simulink model "Homing"  (R2025b)
settings: Solver=FixedStepAuto  StartTime=0.0  StopTime=inf  FixedStep=Ts  RelTol=1e-3
model workspace (MATLAB code in the model file):
  | tgName = 'performance4';
values from neighbouring files (symbols this model uses):
  data = rtRun.export    [postProcess.m]
  Ts = 0.001    [initHoming.m]
undefined symbols (not defined in the file or in its folder): drawWire_m, drawWire_mpers, linearPower_W, netForce_N
libraries: slrealtimeethercatlib x11, slrealtimeloglib x3, simulink x3, eeGeneralControl x3, slrealtimeutilitieslib x2, dspstat3 x2, slrealtimeptplib x1, dspsigops x1
settings Model: Creator=Wave User  LastModifiedBy=bosmab
settings SolverCC: ConcurrentTasks=on  PositivePriorityOrder=on
settings OptimizationCC: BlockReduction=off  OptimizeBlockIOStorage=off
settings DebuggingCC: TasksWithSamePriorityMsg=none
settings HardwareCC: ProdBitPerLong=64.0  ProdLongLongMode=on  ProdHWDeviceType=Intel->x86-64 (Linux 64)
settings RTWCC: SystemTargetFile=speedgoat.tlc  TemplateMakefile=slrealtime_default_tmf  RTWVerbose=off  Toolchain=Simulink Real-Time Toolchain  BuildConfiguration=Faster Runs  CodeExecutionProfiling=on  TargetLang=C++  Description=Speedgoat Real-Time Target Machine
settings SimulinkRealTimeTargetCC: SLRTFileLogMaxRuns=1.0  ExtModeMaxTrigDuration=10.0  ExtModeStaticAllocSize=1000000.0  ExtModeTransport=0.0  MultiwordLength=2048.0  DynamicStringBufferSize=256.0  PreserveMATLABNamespacesInGeneratedCode=on  SubcomponentCodeInterfacePackaging=Reusable function  InstructionSetFMA=off  LogToMDFFile=off

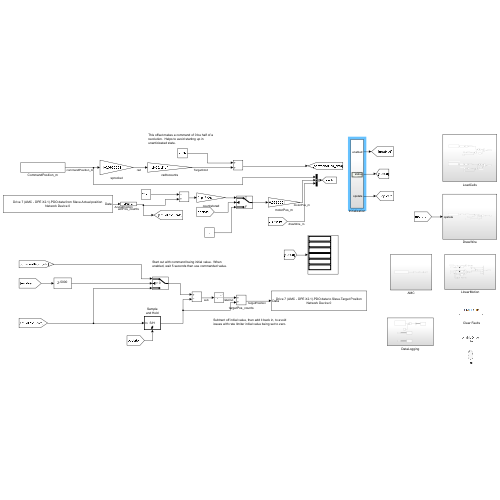
[thumbnail: Simulink's stored preview of the top-level diagram]
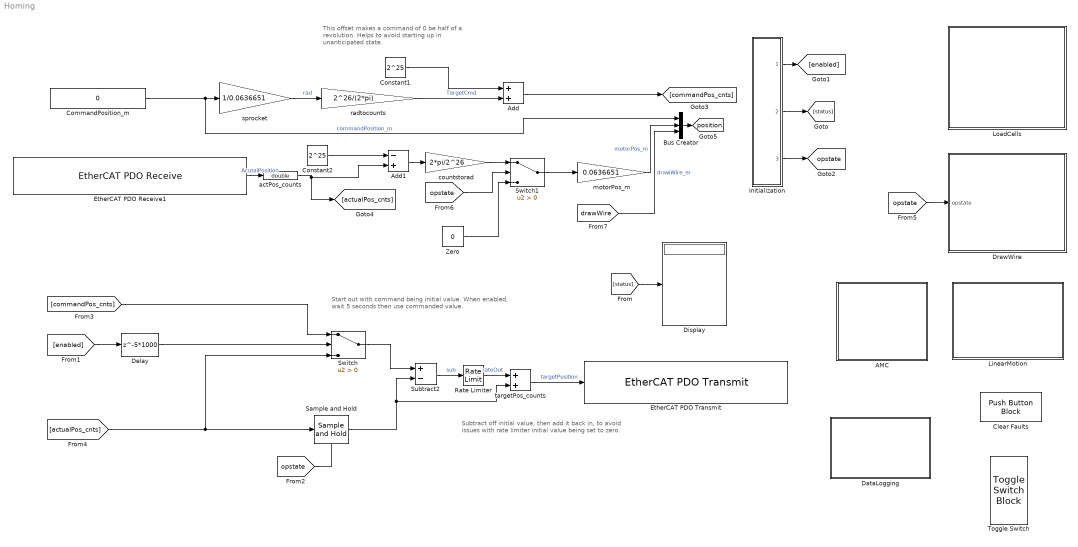
== system Homing ==
  note: Start out with command being initial value. When enabled, wait 5 seconds then use commanded value.
  note: This offset makes a command of 0 be half of a revolution. Helps to avoid starting up in unanticipated state.
  note: Subtract off initial value, then add it back in, to avoid issues with rate limiter initial value being set to zero.
  AMC : Subsystem
  Add : Sum
  Add1 : Sum  Inputs=-+
  Bus Creator : BusCreator  Inputs=3
  Clear Faults : PushButtonBlock  ButtonText=Clear Faults  IconOnColor=[0.0, 0.39215686274509803, 0.0]  IconOffColor=[0.0, 1.0, 0.0]  OffValue=0.000000
  CommandPosition_m : Constant  Value=0  OutDataTypeStr=double
  Constant1 : Constant  Value=2^25  OutDataTypeStr=int32
  Constant2 : Constant  Value=2^25  OutDataTypeStr=double
  DataLogging : Subsystem
  Delay : Delay  DelayLength=5*1000
  Display : Display
  DrawWire : Subsystem
  EtherCAT PDO Receive1 : slrealtimeethercatlib/EtherCAT PDO Receive  Priority=2  sig_name=Drive 7 (AMC - DPE X2.1).PDO data from Slave.Actual position  sig_offset=592  sig_type=int32  type_size=32  sig_dim=1  device_id=0  sample_time=0.001000
  EtherCAT PDO Transmit : slrealtimeethercatlib/EtherCAT PDO Transmit  Priority=3  sig_name=Drive 7 (AMC - DPE X2.1).PDO data to Slave.Target Position  sig_offset=592  sig_type=int32  type_size=32  sig_dim=1  device_id=0  sample_time=0.001000
  Initialization : Subsystem
  LinearMotion : Subsystem
  LoadCells : Subsystem
  Rate Limiter : RateLimiter  RisingSlewLimit=1e6  FallingSlewLimit=-1e6  SampleTimeMode=inherited
  Sample and Hold : dspsigops/Sample and Hold  trig=Rising edge  initCond=0  latchinput=off
  Subtract2 : Sum  Inputs=+-
  Switch : Switch  Criteria=u2 > Threshold  SaturateOnIntegerOverflow=off  InputSameDT=off
  Switch1 : Switch  Criteria=u2 > Threshold  SaturateOnIntegerOverflow=off  InputSameDT=off
  Toggle Switch : ToggleSwitchBlock
  Zero : Constant  Value=0  OutDataTypeStr=Inherit: Inherit via back propagation
  actPos_counts : DataTypeConversion  OutDataTypeStr=double  SaturateOnIntegerOverflow=off  RndMeth=Floor
  countstorad : Gain  Gain=2*pi/2^26  OutDataTypeStr=double
  motorPos_m : Gain  Gain=0.0636651
  radtocounts : Gain  Gain=2^26/(2*pi)  OutDataTypeStr=int32
  sprocket : Gain  Gain=1/0.0636651
  targetPos_counts : Sum  OutDataTypeStr=int32
  tag scope: opstate=global, position=global
  wires:
  Sample and Hold/1 -> Subtract2/2, targetPos_counts/2
  Subtract2/1 -> Rate Limiter/1  "sub"
  Rate Limiter/1 -> targetPos_counts/1  "rateOut"
  targetPos_counts/1 -> EtherCAT PDO Transmit/1  "targetPosition"
  Delay/1 -> Switch/2
  Switch/1 -> Subtract2/1
  [enabled] -> Delay/1
  CommandPosition_m/1 -> Bus Creator/1, sprocket/1  "commandPosition_m"
  sprocket/1 -> radtocounts/1  "rad"
  countstorad/1 -> Switch1/1
  motorPos_m/1 -> Bus Creator/2  "motorPos_m"
  Constant1/1 -> Add/1
  radtocounts/1 -> Add/2  "TargetCmd"
  Add/1 -> [commandPos_cnts]
  EtherCAT PDO Receive1/1 -> actPos_counts/1  "AcutalPosition"
  Constant2/1 -> Add1/1
  Add1/1 -> countstorad/1
  [status] -> Display/1
  Initialization/2(status) -> [status]
  Initialization/1(enabled) -> [enabled]
  Initialization/3(opstate) -> [opstate]
  [opstate] -> Sample and Hold/Trigger
  [commandPos_cnts] -> Switch/1
  [actualPos_cnts] -> Switch/3, Sample and Hold/1
  [opstate] -> DrawWire/1(opstate)
  Zero/1 -> Switch1/3
  [opstate] -> Switch1/2
  Switch1/1 -> motorPos_m/1
  Bus Creator/1 -> [position]
  [drawWire] -> Bus Creator/3  "drawWire_m"
  actPos_counts/1 -> [actualPos_cnts], Add1/2

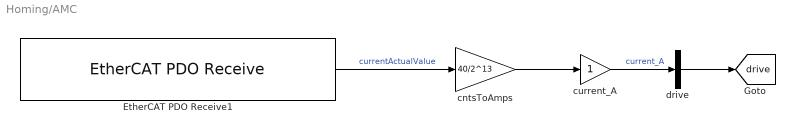
== system Homing/AMC ==
  EtherCAT PDO Receive1 : slrealtimeethercatlib/EtherCAT PDO Receive  Priority=2  sig_name=Drive 7 (AMC - DPE X2.1).PDO data from Slave.Actual Current  sig_offset=656  sig_type=int16  type_size=16  sig_dim=1  device_id=0  sample_time=0.001000
  cntsToAmps : Gain  Gain=40/2^13  OutDataTypeStr=double
  current_A : Gain  OutDataTypeStr=double
  drive : BusCreator  Inputs=1
  tag scope: drive=global
  wires:
  EtherCAT PDO Receive1/1 -> cntsToAmps/1  "currentActualValue"
  drive/1 -> [drive]
  current_A/1 -> drive/1  "current_A"
  cntsToAmps/1 -> current_A/1

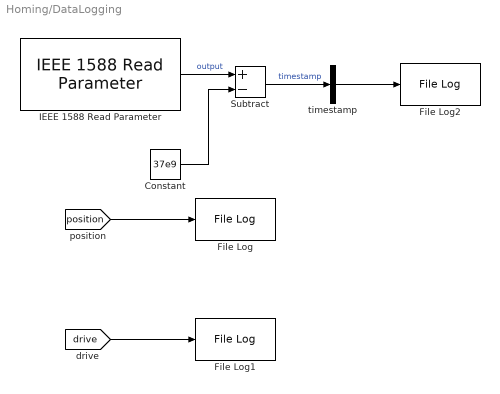
== system Homing/DataLogging ==
  Constant : Constant  Value=37e9  OutDataTypeStr=double
  File Log : slrealtimeloglib/File Log  decimation=1  inputProcessing=Elements as channels (sample based)
  File Log1 : slrealtimeloglib/File Log  decimation=1  inputProcessing=Elements as channels (sample based)
  File Log2 : slrealtimeloglib/File Log  decimation=1  inputProcessing=Elements as channels (sample based)
  IEEE 1588 Read Parameter : slrealtimeptplib/IEEE 1588 Read Parameter  Priority=1  ID=1  param=1. System time (nanosecond)  sample_time=Ts
  Subtract : Sum  Inputs=+-  OutDataTypeStr=double
  timestamp : BusCreator  Inputs=timestamp
  wires:
  [position] -> File Log/1
  [drive] -> File Log1/1
  IEEE 1588 Read Parameter/1 -> Subtract/1  "output"
  Constant/1 -> Subtract/2
  Subtract/1 -> timestamp/1  "timestamp"
  timestamp/1 -> File Log2/1

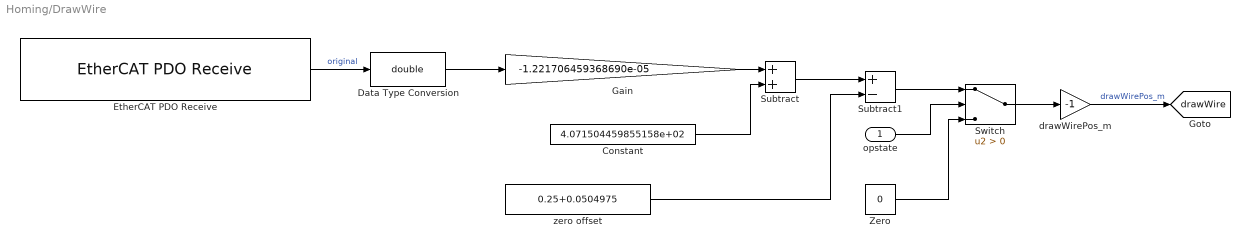
== system Homing/DrawWire ==
  opstate : Inport
  Constant : Constant  Value=4.071504459855158e+02
  Data Type Conversion : DataTypeConversion  OutDataTypeStr=double  SaturateOnIntegerOverflow=off  RndMeth=Floor
  EtherCAT PDO Receive : slrealtimeethercatlib/EtherCAT PDO Receive  Priority=2  sig_name=Term 9 (EL5002).SSI Inputs Channel 1.Counter value  sig_offset=1216  sig_type=uint32  type_size=32  sig_dim=1  device_id=0  sample_time=0.001000
  Gain : Gain  Gain=-1.221706459368690e-05  OutDataTypeStr=double
  Subtract : Sum
  Subtract1 : Sum  Inputs=+-
  Switch : Switch  Criteria=u2 > Threshold  SaturateOnIntegerOverflow=off  InputSameDT=off
  Zero : Constant  Value=0  OutDataTypeStr=Inherit: Inherit via back propagation
  drawWirePos_m : Gain  Gain=-1
  zero offset : Constant  Value=0.25+0.0504975
  tag scope: drawWire=global
  wires:
  Gain/1 -> Subtract/1
  Subtract/1 -> Subtract1/1
  zero offset/1 -> Subtract1/2
  EtherCAT PDO Receive/1 -> Data Type Conversion/1  "original"
  drawWirePos_m/1 -> [drawWire]  "drawWirePos_m"
  Constant/1 -> Subtract/2
  Data Type Conversion/1 -> Gain/1
  Subtract1/1 -> Switch/1
  opstate/1 -> Switch/2
  Switch/1 -> drawWirePos_m/1
  Zero/1 -> Switch/3

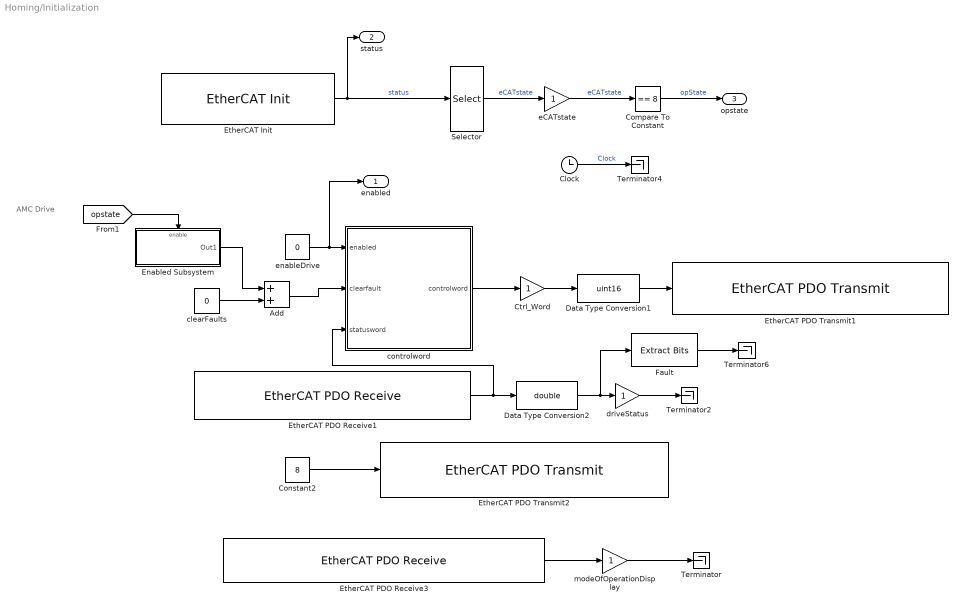
== system Homing/Initialization ==
  note: AMC Drive
  Add : Sum
  Clock : Clock
  Compare To Constant : simulink/Logic and Bit Operations/Compare To Constant  relop===  const=8  OutDataTypeStr=boolean
  Constant2 : Constant  Value=8  OutDataTypeStr=uint16
  Ctrl_Word : Gain
  Data Type Conversion1 : DataTypeConversion  OutDataTypeStr=uint16  SaturateOnIntegerOverflow=off  RndMeth=Floor
  Data Type Conversion2 : DataTypeConversion  OutDataTypeStr=double  SaturateOnIntegerOverflow=off  RndMeth=Floor
  Enabled Subsystem : Subsystem  TreatAsAtomicUnit=on
  EtherCAT Init : slrealtimeethercatlib/EtherCAT Init  Priority=0  config_file=C:\Software\LUPA\Simulink\EtherCAT\LUPAxml.xml  device_id=0  portnum=1  initstate=2  dctuning=0  enaDebug=0  logFile='c:\dbglog.txt'  sample_time=0.001000  DCMode=2
  EtherCAT PDO Receive1 : slrealtimeethercatlib/EtherCAT PDO Receive  Priority=2  sig_name=Drive 7 (AMC - DPE X2.1).PDO data from Slave.Status Word  sig_offset=576  sig_type=uint16  type_size=16  sig_dim=1  device_id=0  sample_time=0.001000
  EtherCAT PDO Receive3 : slrealtimeethercatlib/EtherCAT PDO Receive  Priority=2  sig_name=Drive 7 (AMC - DPE X2.1).PDO data from Slave.Mode Of Operation Display  sig_offset=704  sig_type=uint16  type_size=16  sig_dim=1  device_id=0  sample_time=0.001000
  EtherCAT PDO Transmit1 : slrealtimeethercatlib/EtherCAT PDO Transmit  Priority=3  sig_name=Drive 7 (AMC - DPE X2.1).PDO data to Slave.Control Word  sig_offset=576  sig_type=uint16  type_size=16  sig_dim=1  device_id=0  sample_time=0.001000
  EtherCAT PDO Transmit2 : slrealtimeethercatlib/EtherCAT PDO Transmit  Priority=3  sig_name=Drive 7 (AMC - DPE X2.1).PDO data to Slave.Modes Of Operation  sig_offset=688  sig_type=uint16  type_size=16  sig_dim=1  device_id=0  sample_time=0.001000
  Fault : simulink/Logic and Bit Operations/Extract Bits  bitsToExtract=Range of bits  numBits=8  bitIdxRange=[3]  outScalingMode=Preserve fixed-point scaling
  Selector : Selector  InputPortWidth=6  IndexOptions=Index vector (dialog)  Indices=2  OutputSizes=1
  Terminator{,2,4,6} (4 alike) : Terminator
  clearFaults : Constant  Value=0
  controlword : MATLAB Function  TreatAsAtomicUnit=on
  driveStatus : Gain
  eCATstate : Gain  OutDataTypeStr=double
  enableDrive : Constant  Value=0
  modeOfOperationDisplay : Gain  OutDataTypeStr=double
  enabled : Outport
  status : Outport  Port=2
  opstate : Outport  Port=3
  wires:
  Ctrl_Word/1 -> Data Type Conversion1/1
  enableDrive/1 -> enabled/1, controlword/1(enabled)
  Constant2/1 -> EtherCAT PDO Transmit2/1
  controlword/1(controlword) -> Ctrl_Word/1
  Data Type Conversion2/1 -> Fault/1, driveStatus/1
  EtherCAT PDO Receive1/1 -> Data Type Conversion2/1, controlword/3(statusword)
  Data Type Conversion1/1 -> EtherCAT PDO Transmit1/1
  clearFaults/1 -> Add/2
  driveStatus/1 -> Terminator2/1
  Fault/1 -> Terminator6/1
  Clock/1 -> Terminator4/1  "Clock"
  EtherCAT Init/1 -> status/1, Selector/1  "status"
  eCATstate/1 -> Compare To Constant/1  "eCATstate"
  Selector/1 -> eCATstate/1  "eCATstate"
  Compare To Constant/1 -> opstate/1  "opState"
  EtherCAT PDO Receive3/1 -> modeOfOperationDisplay/1
  modeOfOperationDisplay/1 -> Terminator/1
  Enabled Subsystem/1(Out1) -> Add/1
  [opstate] -> Enabled Subsystem/Enable
  Add/1 -> controlword/2(clearfault)

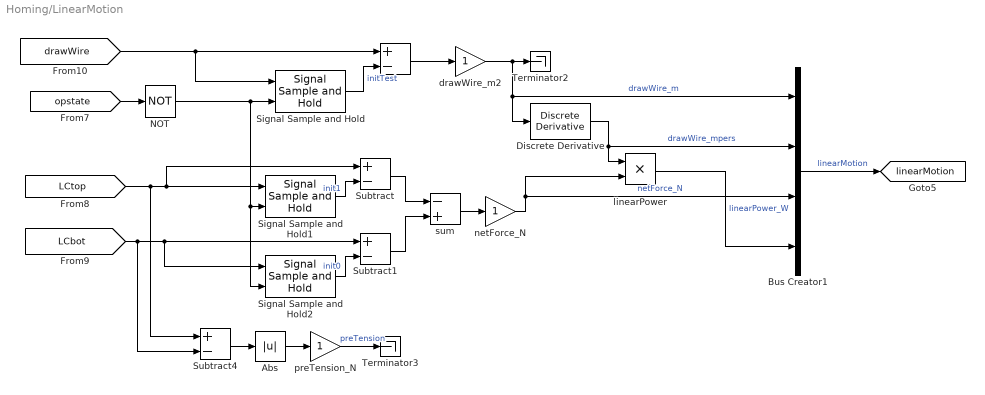
== system Homing/LinearMotion ==
  " " : Sum  Inputs=+-
  Abs : Abs  SaturateOnIntegerOverflow=off
  Bus Creator1 : BusCreator  Inputs=drawWire_m,drawWire_mpers,netForce_N,linearPower_W
  Discrete Derivative : simulink/Discrete/Discrete Derivative  gainval=1.0  ICPrevScaledInput=0.0  OutMin=[]  OutMax=[]  OutDataType=fixdt(1, 16)  OutScaling=2^-10  DoSatur=off
  NOT : Logic  Operator=NOT  IconShape=distinctive  AllPortsSameDT=off  OutDataTypeStr=boolean
  Signal Sample and Hold : eeGeneralControl/Signal Sample and Hold  LabelModeActiveChoice=Discrete  x0=0  Ts=-1
      settings: LibrarySourceBlock=ee_sl_lib/General Control/Signal Sample and Hold
  Signal Sample and Hold1 : eeGeneralControl/Signal Sample and Hold  LabelModeActiveChoice=Discrete  x0=0  Ts=-1
      settings: LibrarySourceBlock=ee_sl_lib/General Control/Signal Sample and Hold
  Signal Sample and Hold2 : eeGeneralControl/Signal Sample and Hold  LabelModeActiveChoice=Discrete  x0=0  Ts=-1
      settings: LibrarySourceBlock=ee_sl_lib/General Control/Signal Sample and Hold
  Subtract : Sum  Inputs=+-
  Subtract1 : Sum  Inputs=+-
  Subtract4 : Sum  Inputs=+-
  Terminator2 : Terminator
  Terminator3 : Terminator
  drawWire_m2 : Gain
  linearPower : Product
  netForce_N : Gain
  preTension_N : Gain
  sum : Sum  Inputs=-+
  tag scope: linearMotion=global
  wires:
  preTension_N/1 -> Terminator3/1  "preTension"
  [drawWire] -> Signal Sample and Hold/1, " "/1
  Subtract4/1 -> Abs/1
  Signal Sample and Hold/1 -> " "/2  "initTest"
  Abs/1 -> preTension_N/1
  [LCtop] -> Subtract4/1, Subtract/1, Signal Sample and Hold1/1
  Subtract1/1 -> sum/2
  netForce_N/1 -> Bus Creator1/3, linearPower/2  "netForce_N"
  " "/1 -> drawWire_m2/1
  Bus Creator1/1 -> [linearMotion]  "linearMotion"
  Signal Sample and Hold1/1 -> Subtract/2  "init1"
  sum/1 -> netForce_N/1
  drawWire_m2/1 -> Bus Creator1/1, Discrete Derivative/1, Terminator2/1  "drawWire_m"
  [LCbot] -> Subtract4/2, Signal Sample and Hold2/1, Subtract1/1
  NOT/1 -> Signal Sample and Hold1/2, Signal Sample and Hold2/2, Signal Sample and Hold/2
  Subtract/1 -> sum/1
  Discrete Derivative/1 -> Bus Creator1/2, linearPower/1  "drawWire_mpers"
  Signal Sample and Hold2/1 -> Subtract1/2  "init0"
  [opstate] -> NOT/1
  linearPower/1 -> Bus Creator1/4  "linearPower_W"

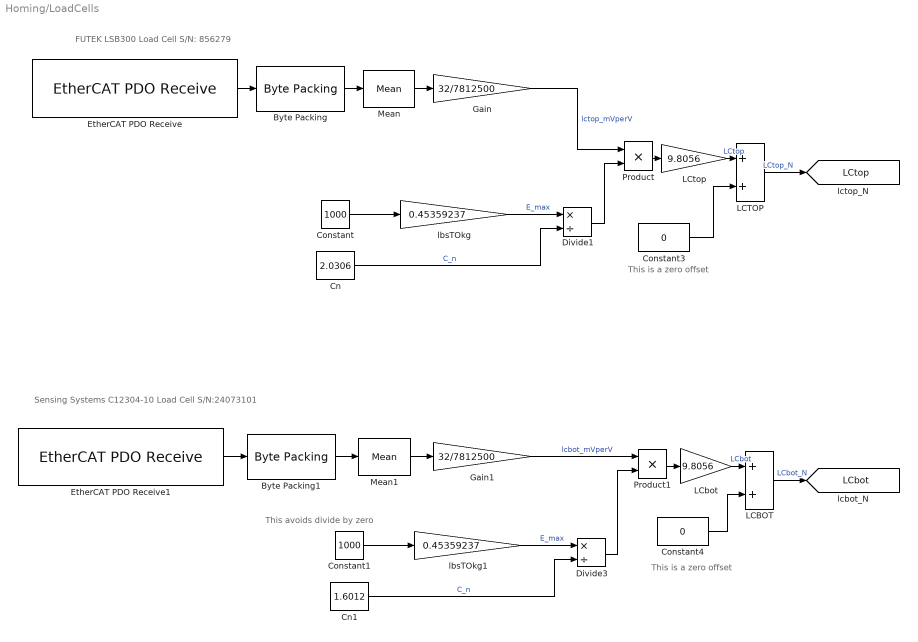
== system Homing/LoadCells ==
  note: FUTEK LSB300 Load Cell S/N: 856279
  note: This is a zero offset
  note: Sensing Systems C12304-10 Load Cell S/N:24073101
  note: This avoids divide by zero
  note: This is a zero offset
  Byte Packing : slrealtimeutilitieslib/Byte Packing  MaskPackedDataType=int32  MaskUnpackedDataTypes={'uint8'}  MaskAlignment=1
  Byte Packing1 : slrealtimeutilitieslib/Byte Packing  MaskPackedDataType=int32  MaskUnpackedDataTypes={'uint8'}  MaskAlignment=1
  Cn : Constant  Value=2.0306
  Cn1 : Constant  Value=1.6012
  Constant : Constant  Value=1000
  Constant1 : Constant  Value=1000
  Constant3 : Constant  Value=0
  Constant4 : Constant  Value=0
  Divide1 : Product  Inputs=*/
  Divide3 : Product  Inputs=*/
  EtherCAT PDO Receive : slrealtimeethercatlib/EtherCAT PDO Receive  Priority=2  sig_name=Term 11 (EL3751).PAI Samples 10.Samples  sig_offset=1744  sig_type=uint8  type_size=8  sig_dim=40  device_id=0  sample_time=0.001000
  EtherCAT PDO Receive1 : slrealtimeethercatlib/EtherCAT PDO Receive  Priority=2  sig_name=Term 10 (EL3751).PAI Samples 10.Samples  sig_offset=1328  sig_type=uint8  type_size=8  sig_dim=40  device_id=0  sample_time=0.001000
  Gain : Gain  Gain=32/7812500
  Gain1 : Gain  Gain=32/7812500
  LCBOT : Sum
  LCTOP : Sum
  LCbot : Gain  Gain=9.8056
  LCtop : Gain  Gain=9.8056
  Mean : dspstat3/Mean  run=off  InputProcessing=Columns as channels (frame based)  reset_popup=None  directionMode=Each column  dimension=1  roiEnable=off  roiType=Rectangles  roiPortion=Entire ROI  roiOutput=Individual statistics for each ROI  roiFlag=off  roundingMode=Floor  overflowMode=off  outputDataTypeStr=Inherit: Same as accumulator  outputMin=[]  outputMax=[]  outputLastDataTypeStr=Inherit: Same as accumulator
  Mean1 : dspstat3/Mean  run=off  InputProcessing=Columns as channels (frame based)  reset_popup=None  directionMode=Each column  dimension=1  roiEnable=off  roiType=Rectangles  roiPortion=Entire ROI  roiOutput=Individual statistics for each ROI  roiFlag=off  roundingMode=Floor  overflowMode=off  outputDataTypeStr=Inherit: Same as accumulator  outputMin=[]  outputMax=[]  outputLastDataTypeStr=Inherit: Same as accumulator
  Product : Product
  Product1 : Product
  lbsTOkg : Gain  Gain=0.45359237
  lbsTOkg1 : Gain  Gain=0.45359237
  tag scope: LCbot=global, LCtop=global
  wires:
  Constant4/1 -> LCBOT/2
  Gain1/1 -> Product1/1  "lcbot_mVperV"
  LCbot/1 -> LCBOT/1  "LCbot"
  Divide1/1 -> Product/2
  Gain/1 -> Product/1  "lctop_mVperV"
  Divide3/1 -> Product1/2
  Constant/1 -> lbsTOkg/1
  LCtop/1 -> LCTOP/1  "LCtop"
  EtherCAT PDO Receive1/1 -> Byte Packing1/1
  Cn1/1 -> Divide3/2  "C_n"
  Constant3/1 -> LCTOP/2
  Product/1 -> LCtop/1
  Mean1/1 -> Gain1/1
  Constant1/1 -> lbsTOkg1/1
  Byte Packing1/1 -> Mean1/1
  Cn/1 -> Divide1/2  "C_n"
  EtherCAT PDO Receive/1 -> Byte Packing/1
  lbsTOkg/1 -> Divide1/1  "E_max"
  LCTOP/1 -> [LCtop]  "LCtop_N"
  LCBOT/1 -> [LCbot]  "LCbot_N"
  Byte Packing/1 -> Mean/1
  lbsTOkg1/1 -> Divide3/1  "E_max"
  Product1/1 -> LCbot/1
  Mean/1 -> Gain/1

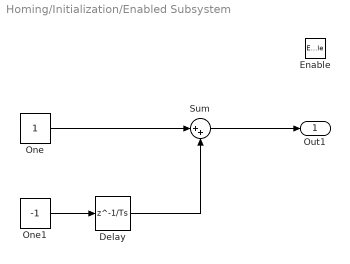
== system Homing/Initialization/Enabled Subsystem ==
  Enable : EnablePort
  Delay : Delay  DelayLength=1/Ts
  One : Constant  OutDataTypeStr=Inherit: Inherit via back propagation
  One1 : Constant  Value=-1  OutDataTypeStr=Inherit: Inherit via back propagation
  Sum : Sum  Inputs=|++
  Out1 : Outport
  wires:
  Sum/1 -> Out1/1
  One/1 -> Sum/1
  One1/1 -> Delay/1
  Delay/1 -> Sum/2

== matlab function Homing/Initialization/controlword ==
  data: enabled input; clearfault input; statusword input; controlword output
function controlword = fcn(enabled, clearfault, statusword)

bitstatus = bitget(statusword,1:16);

if ~clearfault
    if enabled
        if bitstatus(1) == 0 % Ready to switch on not ready
            controlword = 6; % command ready switch on
        elseif ~bitstatus(2) % switched not yet on
            controlword = 7; % command switch on
        elseif ~bitstatus(3) % operation not yet enabled
            controlword = 15; % command enable
        else
            controlword = 15; % maintain enabled state
        end
    else
        controlword = 4; % command disabled
    end
else
    controlword = 128; % command clear faults
end
